simulink model "test01"  (Simulink 4.00)
settings: Solver=FixedStepDiscrete  StartTime=0.0  StopTime=120  FixedStep=1/4000  RelTol=1e-3
settings Model: Creator=root  LastModifiedBy=root  SimulationMode=external  RTWSystemTargetFile=wintarget.tlc  RTWOptions="-aEnforceIntegerDowncast=1 -aExtMode=1 -aFoldNonRolledExpr=1 -aForceParamTrailComments=0 -aGenerateComments=1 -aIgnoreCustomStorageClasses=1 -aIncHierarchyInIds=0 -aInlineInvariantSignals=0 -aInlineParameters=0 -aLocalBlockOutputs=1 -aLogVarNameModifier=\"rt_\" -aRTWVerbose=1 -aRollThreshold=5 -aShowEliminatedStatements=1"  RTWTemplateMakefile=wt_default_tmf  ExtModeAutoUpdateStatusClock=off

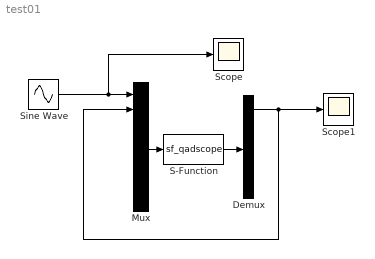
== system test01 ==
  Demux : Demux  Outputs=4  BusSelectionMode=off
  Mux : Mux  Inputs=8
  S-Function : S-Function  FunctionName=sf_qadscope  Parameters=4000  PortCounts=[]  SFunctionModules=''
      settings: OpenFcn=clear all; rtscope
  Scope : Scope
      settings: TimeRange=1  YMin=-5  YMax=5  SaveToWorkspace=off  SaveName=ScopeData  LimitDataPoints=on  MaxDataPoints=5000
  Scope1 : Scope
      settings: TimeRange=1  YMin=-1  YMax=1  SaveToWorkspace=off  LimitDataPoints=on  MaxDataPoints=5000
  Sine Wave : Sin  SineType=Time-based  Amplitude=1  Bias=0  Frequency=2*pi*100  Phase=0  Samples=10  SampleTime=0  Offset=0
  wires:
  Mux/1 -> S-Function/1
  Sine Wave/1 -> Mux/1, Scope/1
  S-Function/1 -> Demux/1
  Demux/1 -> Scope1/1, Mux/2
